simulink model "bitwilse_8"  (R2021a)
settings: Solver=VariableStepAuto  StartTime=0.0  StopTime=10.0  RelTol=1e-3
libraries: simulink x5
settings Model: Creator=yasso  LastModifiedBy=yasso

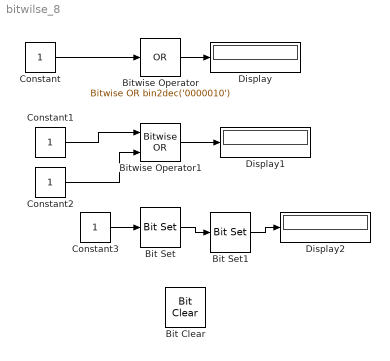
== system bitwilse_8 ==
  Bit Clear : simulink/Logic and Bit Operations/Bit Clear  iBit=0
      settings: SourceProductBaseCode=SL
  Bit Set : simulink/Logic and Bit Operations/Bit Set  iBit=5
      settings: SourceProductBaseCode=SL
  Bit Set1 : simulink/Logic and Bit Operations/Bit Set  iBit=2
      settings: SourceProductBaseCode=SL
  Bitwise Operator : simulink/Logic and Bit Operations/Bitwise Operator  logicop=OR  UseBitMask=on  BitMask=bin2dec('0000010')  BitMaskRealWorld=Stored Integer
  Bitwise Operator1 : simulink/Logic and Bit Operations/Bitwise Operator  logicop=OR  UseBitMask=off  NumInputPorts=2  BitMask=bin2dec('0000010')  BitMaskRealWorld=Stored Integer
  Constant{,1..3} (4 alike) : Constant  OutDataTypeStr=int8
  Display : Display
      settings: Format=binary (Stored Integer)
  Display1 : Display
      settings: Format=binary (Stored Integer)
  Display2 : Display
      settings: Format=binary (Stored Integer)
  wires:
  Bitwise Operator/1 -> Display/1
  Constant/1 -> Bitwise Operator/1
  Constant1/1 -> Bitwise Operator1/1
  Constant2/1 -> Bitwise Operator1/2
  Bitwise Operator1/1 -> Display1/1
  Constant3/1 -> Bit Set/1
  Bit Set/1 -> Bit Set1/1
  Bit Set1/1 -> Display2/1
